simulink model "actuator_models"  (R2024b)
settings: Solver=FixedStepAuto  StartTime=0.0  StopTime=3  FixedStep=0.0001  RelTol=1e-3
libraries: aerolibactuator x1
settings Model: Creator=jonno  LastModifiedBy=jonno

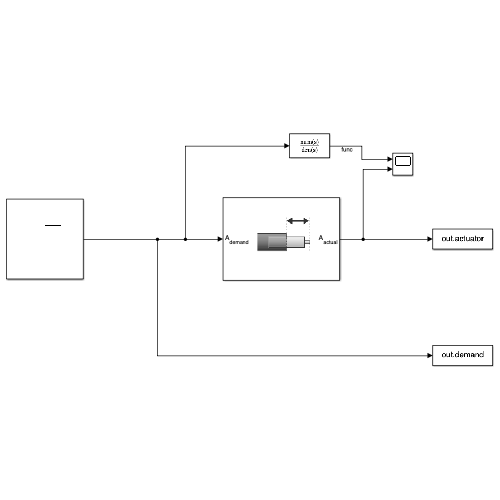
[thumbnail: Simulink's stored preview of the top-level diagram]
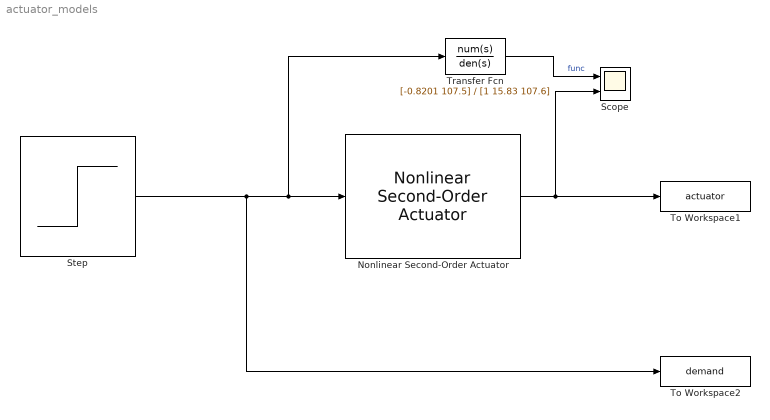
== system actuator_models ==
  Nonlinear Second-Order Actuator : aerolibactuator/Nonlinear Second-Order Actuator  wn_fin=27  z_fin=0.7  fin_max=0.035  fin_min=-0.035  fin_maxrate=0.133  fin_act_0=0  fin_act_vel=0
  Scope : Scope  NumInputPorts=2
  Step : Step  After=0.035  SampleTime=0
  To Workspace1 : ToWorkspace  VariableName=actuator  SaveFormat=Timeseries  SampleTime=-1
  To Workspace2 : ToWorkspace  VariableName=demand  SaveFormat=Timeseries  SampleTime=-1
  Transfer Fcn : TransferFcn  Numerator=[-0.8201 107.5]  Denominator=[1 15.83 107.6]
  wires:
  Step/1 -> To Workspace2/1, Transfer Fcn/1, Nonlinear Second-Order Actuator/1
  Nonlinear Second-Order Actuator/1 -> Scope/2, To Workspace1/1
  Transfer Fcn/1 -> Scope/1  "func"
